simulink subsystem "BatterySystem"  (R2024a)
settings: Solver=VariableStepAuto  StartTime=0.0  StopTime=10  RelTol=1e-3
undefined symbols (not defined in the file): Ion, kWh, Lithium, V
libraries: spsGroundLib x4, spsSeriesRLCBranchLib x3, spsBreakerLib x2, spsMeanLib x2, spsVoltageMeasurementLib x2, spsBatteryLib x1, simulink x1, spsCurrentMeasurementLib x1, slpidlib x1, spsPWMGeneratorDCDCLib x1, spsTwoQuadrantDCDCConverterLib x1
settings Model: DefaultTestHarness=BatterySystem_Harness1  Creator=nakamura  LastModifiedBy=nakamura

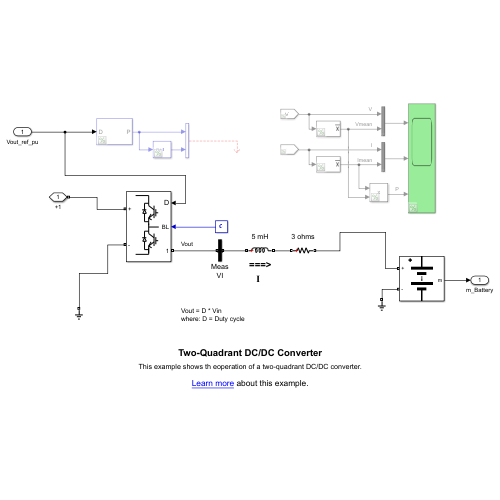
[thumbnail: Simulink's stored preview of the top-level diagram]
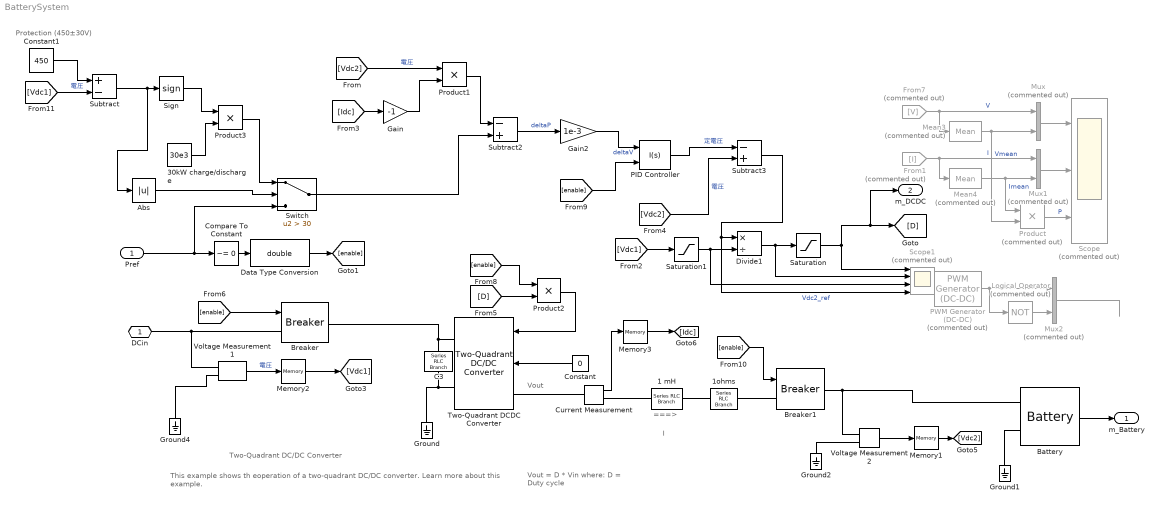
== system BatterySystem ==
  note: Protection (450±30V)
  note: This example shows th eoperation of a two-quadrant DC/DC converter.
      |
      | Learn more about this example.
  note: Vout = D * Vin
      | where: D = Duty cycle
  note: ===>
  note: Two-Quadrant DC/DC Converter
  note: I
  note: Vout
  Pref : Inport
  1 mH : spsSeriesRLCBranchLib/Series RLC Branch  LConnTagsString=__new0  RConnTagsString=__new0  BranchType=L  Resistance=1e-4  Inductance=1e-3  SetiL0=off  InitialCurrent=14  Capacitance=30e-6  Setx0=off  InitialVoltage=150  Measurements=None
  1ohms : spsSeriesRLCBranchLib/Series RLC Branch  LConnTagsString=__new0  RConnTagsString=__new0  BranchType=R  Resistance=0.1  Inductance=750e-6  SetiL0=on  InitialCurrent=14  Capacitance=30e-6  Setx0=off  InitialVoltage=150  Measurements=None
  30kW charge/discharge : Constant  Value=30e3
  Abs : Abs  SaturateOnIntegerOverflow=off
  Battery : spsBatteryLib/Battery  BatType=Lithium-Ion  ShowTempParam=off  ThermalPreset=no  ShowAgeParam=off  NomV=400  NomQ=25e3/400 %kWh/V  SOC=50  Batt_Tr=0.1  PresetModel=off  MaxQ=250  MinV=300  FullV=465.5949  Dis_rate=108.6957  R=0.016  Normal_OP=226.087  expZone="[432.1543      12.28261]"  current=[6.5 13 32.5]  Units=Time  Tci=20  NomT=20  T2=-30  MaxQ2=4.8  FullV2=7.1  Normal_OP2=5.655  expZone2="[6.58           1]"  Rca=0.6  ti=2000  Dp=0  Neq0=0  Tsim=1e6  Ta1=25  Qeol=5.4*0.9  Reol=0.013333*1.2  Char_age=[2.3478, 3]  Dis_age=[2.3478, 10]  N1=1500  N2=10500  N3=1000  N4=1400  Ta2=45  N5=950
  Breaker : spsBreakerLib/Breaker  InitialState=0  SwitchingTimes="[1/60  5/60]"  External=on  BreakerResistance=1e-6  SnubberResistance=1e8  SnubberCapacitance=inf  Measurements=None  MoreParameters=on  NoBreakLoop=off
  Breaker1 : spsBreakerLib/Breaker  InitialState=0  SwitchingTimes="[1/60  5/60]"  External=on  BreakerResistance=1e-6  SnubberResistance=1e8  SnubberCapacitance=inf  Measurements=None  MoreParameters=on  NoBreakLoop=off
  C3 : spsSeriesRLCBranchLib/Series RLC Branch  LConnTagsString=__new0  RConnTagsString=__new0  BranchType=R  Resistance=1e8  Inductance=1.0  SetiL0=off  InitialCurrent=0  Capacitance=75000e-06  Setx0=off  InitialVoltage=0  Measurements=None
  Compare To Constant : simulink/Logic and Bit Operations/Compare To Constant  relop=~=  const=0  OutDataTypeStr=uint8
  Constant : Constant  Value=0
  Constant1 : Constant  Value=450
  Current Measurement : spsCurrentMeasurementLib/Current Measurement  PhasorSimulation=off  OutputType=Complex  PSBequivalent=0
  Data Type Conversion : DataTypeConversion  OutDataTypeStr=double  SaturateOnIntegerOverflow=off  RndMeth=Floor
  Divide1 : Product  Inputs=*/
  From1 : From  Commented=on  GotoTag=I  TagVisibility=global
  From7 : From  Commented=on  GotoTag=V  TagVisibility=global
  Gain : Gain  Gain=-1
  Gain2 : Gain  Gain=1e-3
  Ground{,1..2,4} (4 alike) : spsGroundLib/Ground  LConnTagsString=a
  Logical Operator : Logic  Commented=on  Operator=NOT  AllPortsSameDT=off  OutDataTypeStr=float('double')
  Mean3 : spsMeanLib/Mean  Commented=on  Freq=1000  Vinit=0  Ts=0
  Mean4 : spsMeanLib/Mean  Commented=on  Freq=1000  Vinit=0  Ts=0
  Memory1 : Memory  InitialCondition=400
  Memory2 : Memory  InitialCondition=400
  Memory3 : Memory
  Mux : Mux  Commented=on  Inputs=2
  Mux1 : Mux  Commented=on  Inputs=2
  Mux2 : Mux  Commented=on  Inputs=2
  PID Controller : slpidlib/PID Controller  Controller=I  Form=Parallel  TimeDomain=Continuous-time  UseExternalTs=off  SampleTime=-1  IntegratorMethod=Forward Euler  FilterMethod=Forward Euler  ControllerParametersSource=internal  P=1  I=10  UseKiTs=off  D=0  UseExternalDerivativeSource=off  N=100  UseFilter=on  TunerSelectOption=Transfer Function Based (PID Tuner App)  InitialConditionSource=internal  InitialConditionForIntegrator=0  InitialConditionForFilter=0  DifferentiatorICPrevScaledInput=0  ExternalReset=either  TrackingMode=off  Kt=1  LimitOutput=on  SatLimitsSource=internal  UpperSaturationLimit=20  LowerSaturationLimit=-20  LinearizeAsGain=on  AntiWindupMode=none  Kb=1  LimitIntegrator=off  UpperIntegratorSaturationLimit=inf  LowerIntegratorSaturationLimit=-inf  POutMin=[]  POutMax=[]  IOutMin=[]  IOutMax=[]  DOutMin=[]  DOutMax=[]  NOutMin=[]  NOutMax=[]  SumOutMin=[]  SumOutMax=[]  SaturationOutMin=[]  SaturationOutMax=[]  PParamMin=[]  PParamMax=[]  IParamMin=[]  IParamMax=[]  DParamMin=[]  DParamMax=[]  NParamMin=[]  NParamMax=[]  KbParamMin=[]  KbParamMax=[]  KtParamMin=[]  KtParamMax=[]  KbOutMin=[]  KbOutMax=[]  KtOutMin=[]  KtOutMax=[]  IntegratorOutMin=[]  IntegratorOutMax=[]  FilterOutMin=[]  FilterOutMax=[]  SumI1OutMin=[]  SumI1OutMax=[]  SumI2OutMin=[]  SumI2OutMax=[]  SumI3OutMin=[]  SumI3OutMax=[]  SumI4OutMin=[]  SumI4OutMax=[]  SumDOutMin=[]  SumDOutMax=[]  DifferentiatorOutMin=[]  DifferentiatorOutMax=[]  FilterDiffOutCoefMin=[]  FilterDiffOutCoefMax=[]  ReciprocalOutMin=[]  ReciprocalOutMax=[]  SumDenOutMin=[]  SumDenOutMax=[]  SumNumOutMin=[]  SumNumOutMax=[]  DivideOutMin=[]  DivideOutMax=[]  UdiffTsProdOutMin=[]  UdiffTsProdOutMax=[]  NTsProdOutMin=[]  NTsProdOutMax=[]  UintegralTsProdOutMin=[]  UintegralTsProdOutMax=[]  UngainTsProdOutMin=[]  UngainTsProdOutMax=[]  ClampingZeroOutDataTypeStr=Inherit: Inherit via back propagation  ClampingZeroOutMin=[]  ClampingZeroOutMax=[]  FilterDenConstantOutDataTypeStr=Inherit: Inherit via back propagation  FilterDenConstantOutMin=[]  FilterDenConstantOutMax=[]  PCopyOutDataTypeStr=Inherit: Inherit via back propagation  PCopyOutMin=[]  PCopyOutMax=[]  NCopyOutDataTypeStr=Inherit: Inherit via back propagation  NCopyOutMin=[]  NCopyOutMax=[]  IntegratorContinuousStateAttributes=''  IntegratorStateMustResolveToSignalObject=off  IntegratorRTWStateStorageClass=Auto  FilterContinuousStateAttributes=''  FilterStateMustResolveToSignalObject=off  FilterRTWStateStorageClass=Auto  ParallelPVariant=Disabled  IdealPVariant=Disabled  IVariant=InternalParameters  DVariant=Disabled  IntegratorVariant=Continuous  SatVariant=Enabled  AWVariant=Passthrough  PCopyVariant=Disabled  TRVariant=Disabled  FdbkBlocksVariant=Forward  IdealPFdbkVariant=Disabled  SatFdbkVariant=Disabled  DerivativeFilterVariant=Disabled  NVariant=Disabled  NCopyVariant=Disabled_SignalSpec  FilterICVariant=Disabled  IntegratorICVariant=InternalICs  ExternalResetVariant=ExternalReset  TRSumVariant=Passthrough  SumFdbkVariant=Disabled  SumVariant=Passthrough_I  TsampFilterVariant=InternalTs  TsampNgainVariant=Passthrough  TsampIntegralVariant=Disabled_SignalSpec  ExternalSaturationOutDataTypeStr=Inherit: Same as second input  DerivativeSourceVariant=Disabled
  PWM Generator (DC-DC) : spsPWMGeneratorDCDCLib/PWM Generator (DC-DC)  Commented=on  Fsw=2e3  Ts=0
  Product : Product  Commented=on
  Product1 : Product
  Product2 : Product
  Product3 : Product
  Saturation : Saturate  UpperLimit=1  LowerLimit=0.5
  Saturation1 : Saturate  UpperLimit=inf  LowerLimit=1
  Scope : Scope  Commented=on  NumInputPorts=3
  Scope1 : Scope  Commented=on  NumInputPorts=4
  Sign : Signum
  Subtract : Sum  Inputs=+-
  Subtract2 : Sum  Inputs=-+
  Subtract3 : Sum  Inputs=-+
  Switch : Switch  Criteria=u2 > Threshold  Threshold=30  SaturateOnIntegerOverflow=off  InputSameDT=off
  Two-Quadrant DCDC Converter : spsTwoQuadrantDCDCConverterLib/Two-Quadrant DC//DC Converter  ModelType=Average model (D-controlled)  Ron=1e-3  Rs=1e6  Cs=inf  Vforward=[0,0]  Ron_Diode=1e-6  Rs_Diode=1e6  Cs_Diode=inf  Vf_Diode=1e-6  Rs_CurrentSource=inf  Ron_ACsource=1e-3
      settings: LibrarySourceBlock=|
      | sps_lib/Power Electronics/Two-Quadrant
      | DC//DC Converter
  Voltage Measurement1 : spsVoltageMeasurementLib/Voltage Measurement  PhasorSimulation=off  OutputType=Complex  PSBequivalent=0
  Voltage Measurement2 : spsVoltageMeasurementLib/Voltage Measurement  Tag=PoWeRsYsTeMmEaSuReMeNt  PhasorSimulation=off  OutputType=Magnitude  PSBequivalent=0
  DCin : PMIOPort  Side=Left
  m_Battery : Outport
  m_DCDC : Outport  Port=2
  wires:
  PWM Generator (DC-DC)/1 -> Logical Operator/1, Mux2/1
  From1/1 -> Mux1/1, Mean4/1  "I"
  Logical Operator/1 -> Mux2/2
  Mux1/1 -> Scope/2
  Mean3/1 -> Product/2, Mux/2  "Vmean"
  Mean4/1 -> Product/1, Mux1/2  "Imean"
  Product/1 -> Scope/3  "P"
  Mux2/1 -> ?
  Constant/1 -> Two-Quadrant DCDC Converter/2
  From7/1 -> Mean3/1, Mux/1  "V"
  Mux/1 -> Scope/1
  Battery/1 -> m_Battery/1
  PID Controller/1 -> Subtract3/1  "定電圧"
  Subtract3/1 -> Divide1/1, Scope1/4  "Vdc2_ref"
  Product1/1 -> Subtract2/1
  Saturation1/1 -> Scope1/3, Divide1/2
  Divide1/1 -> Saturation/1, Scope1/2
  [Vdc2] -> Product1/1  "電圧"
  Subtract2/1 -> Gain2/1  "deltaP"
  [Vdc2] -> Subtract3/2  "電圧"
  [D] -> Product2/2
  Current Measurement/1 -> Memory3/1
  Memory3/1 -> [Idc]
  Gain/1 -> Product1/2
  [Idc] -> Gain/1
  Gain2/1 -> PID Controller/1  "deltaV"
  Pref/1 -> Compare To Constant/1, Switch/3
  Product2/1 -> Two-Quadrant DCDC Converter/1
  Compare To Constant/1 -> Data Type Conversion/1
  [enable] -> Breaker/1
  [enable] -> Product2/1
  [enable] -> PID Controller/2
  [enable] -> Breaker1/1
  Data Type Conversion/1 -> [enable]
  [Vdc1] -> Saturation1/1
  Saturation/1 -> Scope1/1, [D], m_DCDC/1
  Voltage Measurement2/1 -> Memory1/1
  Memory1/1 -> [Vdc2]
  Voltage Measurement1/1 -> Memory2/1  "電圧"
  Memory2/1 -> [Vdc1]
  [Vdc1] -> Subtract/2  "電圧"
  Switch/1 -> Subtract2/2
  Product3/1 -> Switch/1
  Constant1/1 -> Subtract/1
  Subtract/1 -> Abs/1, Sign/1
  Abs/1 -> Switch/2
  Sign/1 -> Product3/1
  30kW charge/discharge/1 -> Product3/2
  connections:
  Battery/LConn1 -- Voltage Measurement2/LConn1 -- Breaker1/RConn1
  Two-Quadrant DCDC Converter/RConn2 -- C3/RConn1 -- Ground/LConn1
  Breaker/LConn1 -- DCin/RConn1 -- Voltage Measurement1/LConn1
  C3/LConn1 -- Two-Quadrant DCDC Converter/RConn1 -- Breaker/RConn1
  Current Measurement/LConn1 -- Two-Quadrant DCDC Converter/LConn1
  1 mH/RConn1 -- 1ohms/LConn1
  Current Measurement/RConn1 -- 1 mH/LConn1
  Battery/LConn2 -- Ground1/LConn1
  Breaker1/LConn1 -- 1ohms/RConn1
  Ground2/LConn1 -- Voltage Measurement2/LConn2
  Ground4/LConn1 -- Voltage Measurement1/LConn2
